simulink model "gm_parallel_phase_voltages_per_switching_state_6_vnl"  (R2022a)
settings: Solver=FixedStepDiscrete  StartTime=0.0  StopTime=10.0  RelTol=1e-3
undefined symbols (not defined in the file or in its folder): f_c, Rt, u_dc
libraries: hdlmdlgenlib x82, simulink x6, hdlsllib x2
(part 6 of 7)

== system gm_parallel_phase_voltages_per_switching_state_6_vnl/Phase_voltages_per_switching_state/Subsystem/MATLAB Function5/adder2 ==
  In1 : Inport
  In2 : Inport  Port=2
  adder2 : Sum  OutDataTypeStr=single  SampleTime=1e-08
  adder2_pd1 : Delay  DelayLength=6
  Out1 : Outport
  wires:
  adder2_pd1/1 -> Out1/1
  adder2/1 -> adder2_pd1/1
  In2/1 -> adder2/2
  In1/1 -> adder2/1

== system gm_parallel_phase_voltages_per_switching_state_6_vnl/Phase_voltages_per_switching_state/Subsystem/MATLAB Function5/cos_to_sincos ==
  In1 : Inport
  cos_to_sincos : Trigonometry  Operator=sincos  SampleTime=1e-08
  cos_to_sincos_pd1 : Delay  DelayLength=27
  cos_to_sincos_pd2 : Delay  DelayLength=27
  Out1 : Outport
  Out2 : Outport  Port=2
  wires:
  cos_to_sincos_pd2/1 -> Out2/1
  cos_to_sincos/2 -> cos_to_sincos_pd2/1
  cos_to_sincos_pd1/1 -> Out1/1
  cos_to_sincos/1 -> cos_to_sincos_pd1/1
  In1/1 -> cos_to_sincos/1

== system gm_parallel_phase_voltages_per_switching_state_6_vnl/Phase_voltages_per_switching_state/Subsystem/MATLAB Function5/multiplier ==
  In1 : Inport
  In2 : Inport  Port=2
  multiplier : Product  Inputs=**  OutDataTypeStr=single  SampleTime=1e-08
  multiplier_pd1 : Delay  DelayLength=6
  Out1 : Outport
  wires:
  multiplier_pd1/1 -> Out1/1
  multiplier/1 -> multiplier_pd1/1
  In2/1 -> multiplier/2
  In1/1 -> multiplier/1

== system gm_parallel_phase_voltages_per_switching_state_6_vnl/Phase_voltages_per_switching_state/Subsystem/MATLAB Function5/multiplier1 ==
  In1 : Inport
  In2 : Inport  Port=2
  multiplier1 : Product  Inputs=**  OutDataTypeStr=single  SampleTime=1e-08
  multiplier1_pd1 : Delay  DelayLength=6
  Out1 : Outport
  wires:
  multiplier1_pd1/1 -> Out1/1
  multiplier1/1 -> multiplier1_pd1/1
  In2/1 -> multiplier1/2
  In1/1 -> multiplier1/1

== system gm_parallel_phase_voltages_per_switching_state_6_vnl/Phase_voltages_per_switching_state/Subsystem/MATLAB Function5/multiplier2 ==
  In1 : Inport
  In2 : Inport  Port=2
  multiplier2 : Product  Inputs=**  OutDataTypeStr=single  SampleTime=1e-08
  multiplier2_pd1 : Delay  DelayLength=6
  Out1 : Outport
  wires:
  multiplier2_pd1/1 -> Out1/1
  multiplier2/1 -> multiplier2_pd1/1
  In2/1 -> multiplier2/2
  In1/1 -> multiplier2/1

== system gm_parallel_phase_voltages_per_switching_state_6_vnl/Phase_voltages_per_switching_state/Subsystem/MATLAB Function5/multiplier3 ==
  In1 : Inport
  In2 : Inport  Port=2
  multiplier3 : Product  Inputs=**  OutDataTypeStr=single  SampleTime=1e-08
  multiplier3_pd1 : Delay  DelayLength=6
  Out1 : Outport
  wires:
  multiplier3_pd1/1 -> Out1/1
  multiplier3/1 -> multiplier3_pd1/1
  In2/1 -> multiplier3/2
  In1/1 -> multiplier3/1

== system gm_parallel_phase_voltages_per_switching_state_6_vnl/Phase_voltages_per_switching_state/Subsystem/MATLAB Function5/multiplier4 ==
  In1 : Inport
  In2 : Inport  Port=2
  multiplier4 : Product  Inputs=**  OutDataTypeStr=single  SampleTime=1e-08
  multiplier4_pd1 : Delay  DelayLength=6
  Out1 : Outport
  wires:
  multiplier4_pd1/1 -> Out1/1
  multiplier4/1 -> multiplier4_pd1/1
  In2/1 -> multiplier4/2
  In1/1 -> multiplier4/1

== system gm_parallel_phase_voltages_per_switching_state_6_vnl/Phase_voltages_per_switching_state/Subsystem/MATLAB Function5/uminus ==
  In1 : Inport
  uminus : UnaryMinus  SampleTime=1e-08
  Out1 : Outport
  wires:
  uminus/1 -> Out1/1
  In1/1 -> uminus/1

== system gm_parallel_phase_voltages_per_switching_state_6_vnl/Phase_voltages_per_switching_state/Subsystem/MATLAB Function6/adder1 ==
  In1 : Inport
  In2 : Inport  Port=2
  adder1 : Sum  OutDataTypeStr=single  SampleTime=1e-08
  adder1_pd1 : Delay  DelayLength=6
  Out1 : Outport
  wires:
  adder1_pd1/1 -> Out1/1
  adder1/1 -> adder1_pd1/1
  In2/1 -> adder1/2
  In1/1 -> adder1/1

== system gm_parallel_phase_voltages_per_switching_state_6_vnl/Phase_voltages_per_switching_state/Subsystem/MATLAB Function6/adder2 ==
  In1 : Inport
  In2 : Inport  Port=2
  adder2 : Sum  OutDataTypeStr=single  SampleTime=1e-08
  adder2_pd1 : Delay  DelayLength=6
  Out1 : Outport
  wires:
  adder2_pd1/1 -> Out1/1
  adder2/1 -> adder2_pd1/1
  In2/1 -> adder2/2
  In1/1 -> adder2/1

== system gm_parallel_phase_voltages_per_switching_state_6_vnl/Phase_voltages_per_switching_state/Subsystem/MATLAB Function6/cos_to_sincos ==
  In1 : Inport
  cos_to_sincos : Trigonometry  Operator=sincos  SampleTime=1e-08
  cos_to_sincos_pd1 : Delay  DelayLength=27
  cos_to_sincos_pd2 : Delay  DelayLength=27
  Out1 : Outport
  Out2 : Outport  Port=2
  wires:
  cos_to_sincos_pd2/1 -> Out2/1
  cos_to_sincos/2 -> cos_to_sincos_pd2/1
  cos_to_sincos_pd1/1 -> Out1/1
  cos_to_sincos/1 -> cos_to_sincos_pd1/1
  In1/1 -> cos_to_sincos/1

== system gm_parallel_phase_voltages_per_switching_state_6_vnl/Phase_voltages_per_switching_state/Subsystem/MATLAB Function6/multiplier ==
  In1 : Inport
  In2 : Inport  Port=2
  multiplier : Product  Inputs=**  OutDataTypeStr=single  SampleTime=1e-08
  multiplier_pd1 : Delay  DelayLength=6
  Out1 : Outport
  wires:
  multiplier_pd1/1 -> Out1/1
  multiplier/1 -> multiplier_pd1/1
  In2/1 -> multiplier/2
  In1/1 -> multiplier/1

== system gm_parallel_phase_voltages_per_switching_state_6_vnl/Phase_voltages_per_switching_state/Subsystem/MATLAB Function6/multiplier1 ==
  In1 : Inport
  In2 : Inport  Port=2
  multiplier1 : Product  Inputs=**  OutDataTypeStr=single  SampleTime=1e-08
  multiplier1_pd1 : Delay  DelayLength=6
  Out1 : Outport
  wires:
  multiplier1_pd1/1 -> Out1/1
  multiplier1/1 -> multiplier1_pd1/1
  In2/1 -> multiplier1/2
  In1/1 -> multiplier1/1

== system gm_parallel_phase_voltages_per_switching_state_6_vnl/Phase_voltages_per_switching_state/Subsystem/MATLAB Function6/multiplier2 ==
  In1 : Inport
  In2 : Inport  Port=2
  multiplier2 : Product  Inputs=**  OutDataTypeStr=single  SampleTime=1e-08
  multiplier2_pd1 : Delay  DelayLength=6
  Out1 : Outport
  wires:
  multiplier2_pd1/1 -> Out1/1
  multiplier2/1 -> multiplier2_pd1/1
  In2/1 -> multiplier2/2
  In1/1 -> multiplier2/1

== system gm_parallel_phase_voltages_per_switching_state_6_vnl/Phase_voltages_per_switching_state/Subsystem/MATLAB Function6/multiplier3 ==
  In1 : Inport
  In2 : Inport  Port=2
  multiplier3 : Product  Inputs=**  OutDataTypeStr=single  SampleTime=1e-08
  multiplier3_pd1 : Delay  DelayLength=6
  Out1 : Outport
  wires:
  multiplier3_pd1/1 -> Out1/1
  multiplier3/1 -> multiplier3_pd1/1
  In2/1 -> multiplier3/2
  In1/1 -> multiplier3/1

== system gm_parallel_phase_voltages_per_switching_state_6_vnl/Phase_voltages_per_switching_state/Subsystem/MATLAB Function6/multiplier4 ==
  In1 : Inport
  In2 : Inport  Port=2
  multiplier4 : Product  Inputs=**  OutDataTypeStr=single  SampleTime=1e-08
  multiplier4_pd1 : Delay  DelayLength=6
  Out1 : Outport
  wires:
  multiplier4_pd1/1 -> Out1/1
  multiplier4/1 -> multiplier4_pd1/1
  In2/1 -> multiplier4/2
  In1/1 -> multiplier4/1

== system gm_parallel_phase_voltages_per_switching_state_6_vnl/Phase_voltages_per_switching_state/Subsystem/MATLAB Function6/uminus ==
  In1 : Inport
  uminus : UnaryMinus  SampleTime=1e-08
  Out1 : Outport
  wires:
  uminus/1 -> Out1/1
  In1/1 -> uminus/1

== system gm_parallel_phase_voltages_per_switching_state_6_vnl/Phase_voltages_per_switching_state/Subsystem/MATLAB Function7/adder1 ==
  In1 : Inport
  In2 : Inport  Port=2
  adder1 : Sum  OutDataTypeStr=single  SampleTime=1e-08
  adder1_pd1 : Delay  DelayLength=6
  Out1 : Outport
  wires:
  adder1_pd1/1 -> Out1/1
  adder1/1 -> adder1_pd1/1
  In2/1 -> adder1/2
  In1/1 -> adder1/1

== system gm_parallel_phase_voltages_per_switching_state_6_vnl/Phase_voltages_per_switching_state/Subsystem/MATLAB Function7/adder2 ==
  In1 : Inport
  In2 : Inport  Port=2
  adder2 : Sum  OutDataTypeStr=single  SampleTime=1e-08
  adder2_pd1 : Delay  DelayLength=6
  Out1 : Outport
  wires:
  adder2_pd1/1 -> Out1/1
  adder2/1 -> adder2_pd1/1
  In2/1 -> adder2/2
  In1/1 -> adder2/1

== system gm_parallel_phase_voltages_per_switching_state_6_vnl/Phase_voltages_per_switching_state/Subsystem/MATLAB Function7/cos_to_sincos ==
  In1 : Inport
  cos_to_sincos : Trigonometry  Operator=sincos  SampleTime=1e-08
  cos_to_sincos_pd1 : Delay  DelayLength=27
  cos_to_sincos_pd2 : Delay  DelayLength=27
  Out1 : Outport
  Out2 : Outport  Port=2
  wires:
  cos_to_sincos_pd2/1 -> Out2/1
  cos_to_sincos/2 -> cos_to_sincos_pd2/1
  cos_to_sincos_pd1/1 -> Out1/1
  cos_to_sincos/1 -> cos_to_sincos_pd1/1
  In1/1 -> cos_to_sincos/1

== system gm_parallel_phase_voltages_per_switching_state_6_vnl/Phase_voltages_per_switching_state/Subsystem/MATLAB Function7/multiplier ==
  In1 : Inport
  In2 : Inport  Port=2
  multiplier : Product  Inputs=**  OutDataTypeStr=single  SampleTime=1e-08
  multiplier_pd1 : Delay  DelayLength=6
  Out1 : Outport
  wires:
  multiplier_pd1/1 -> Out1/1
  multiplier/1 -> multiplier_pd1/1
  In2/1 -> multiplier/2
  In1/1 -> multiplier/1

== system gm_parallel_phase_voltages_per_switching_state_6_vnl/Phase_voltages_per_switching_state/Subsystem/MATLAB Function7/multiplier1 ==
  In1 : Inport
  In2 : Inport  Port=2
  multiplier1 : Product  Inputs=**  OutDataTypeStr=single  SampleTime=1e-08
  multiplier1_pd1 : Delay  DelayLength=6
  Out1 : Outport
  wires:
  multiplier1_pd1/1 -> Out1/1
  multiplier1/1 -> multiplier1_pd1/1
  In2/1 -> multiplier1/2
  In1/1 -> multiplier1/1

== system gm_parallel_phase_voltages_per_switching_state_6_vnl/Phase_voltages_per_switching_state/Subsystem/MATLAB Function7/multiplier2 ==
  In1 : Inport
  In2 : Inport  Port=2
  multiplier2 : Product  Inputs=**  OutDataTypeStr=single  SampleTime=1e-08
  multiplier2_pd1 : Delay  DelayLength=6
  Out1 : Outport
  wires:
  multiplier2_pd1/1 -> Out1/1
  multiplier2/1 -> multiplier2_pd1/1
  In2/1 -> multiplier2/2
  In1/1 -> multiplier2/1

== system gm_parallel_phase_voltages_per_switching_state_6_vnl/Phase_voltages_per_switching_state/Subsystem/MATLAB Function7/multiplier3 ==
  In1 : Inport
  In2 : Inport  Port=2
  multiplier3 : Product  Inputs=**  OutDataTypeStr=single  SampleTime=1e-08
  multiplier3_pd1 : Delay  DelayLength=6
  Out1 : Outport
  wires:
  multiplier3_pd1/1 -> Out1/1
  multiplier3/1 -> multiplier3_pd1/1
  In2/1 -> multiplier3/2
  In1/1 -> multiplier3/1

== system gm_parallel_phase_voltages_per_switching_state_6_vnl/Phase_voltages_per_switching_state/Subsystem/MATLAB Function7/multiplier4 ==
  In1 : Inport
  In2 : Inport  Port=2
  multiplier4 : Product  Inputs=**  OutDataTypeStr=single  SampleTime=1e-08
  multiplier4_pd1 : Delay  DelayLength=6
  Out1 : Outport
  wires:
  multiplier4_pd1/1 -> Out1/1
  multiplier4/1 -> multiplier4_pd1/1
  In2/1 -> multiplier4/2
  In1/1 -> multiplier4/1

== system gm_parallel_phase_voltages_per_switching_state_6_vnl/Phase_voltages_per_switching_state/Subsystem/MATLAB Function7/uminus ==
  In1 : Inport
  uminus : UnaryMinus  SampleTime=1e-08
  Out1 : Outport
  wires:
  uminus/1 -> Out1/1
  In1/1 -> uminus/1

== system gm_parallel_phase_voltages_per_switching_state_6_vnl/Phase_voltages_per_switching_state/Subsystem/MATLAB Function8/adder1 ==
  In1 : Inport
  In2 : Inport  Port=2
  adder1 : Sum  OutDataTypeStr=single  SampleTime=1e-08
  adder1_pd1 : Delay  DelayLength=6
  Out1 : Outport
  wires:
  adder1_pd1/1 -> Out1/1
  adder1/1 -> adder1_pd1/1
  In2/1 -> adder1/2
  In1/1 -> adder1/1

== system gm_parallel_phase_voltages_per_switching_state_6_vnl/Phase_voltages_per_switching_state/Subsystem/MATLAB Function8/adder2 ==
  In1 : Inport
  In2 : Inport  Port=2
  adder2 : Sum  OutDataTypeStr=single  SampleTime=1e-08
  adder2_pd1 : Delay  DelayLength=6
  Out1 : Outport
  wires:
  adder2_pd1/1 -> Out1/1
  adder2/1 -> adder2_pd1/1
  In2/1 -> adder2/2
  In1/1 -> adder2/1

== system gm_parallel_phase_voltages_per_switching_state_6_vnl/Phase_voltages_per_switching_state/Subsystem/MATLAB Function8/cos_to_sincos ==
  In1 : Inport
  cos_to_sincos : Trigonometry  Operator=sincos  SampleTime=1e-08
  cos_to_sincos_pd1 : Delay  DelayLength=27
  cos_to_sincos_pd2 : Delay  DelayLength=27
  Out1 : Outport
  Out2 : Outport  Port=2
  wires:
  cos_to_sincos_pd2/1 -> Out2/1
  cos_to_sincos/2 -> cos_to_sincos_pd2/1
  cos_to_sincos_pd1/1 -> Out1/1
  cos_to_sincos/1 -> cos_to_sincos_pd1/1
  In1/1 -> cos_to_sincos/1

== system gm_parallel_phase_voltages_per_switching_state_6_vnl/Phase_voltages_per_switching_state/Subsystem/MATLAB Function8/multiplier ==
  In1 : Inport
  In2 : Inport  Port=2
  multiplier : Product  Inputs=**  OutDataTypeStr=single  SampleTime=1e-08
  multiplier_pd1 : Delay  DelayLength=6
  Out1 : Outport
  wires:
  multiplier_pd1/1 -> Out1/1
  multiplier/1 -> multiplier_pd1/1
  In2/1 -> multiplier/2
  In1/1 -> multiplier/1

== system gm_parallel_phase_voltages_per_switching_state_6_vnl/Phase_voltages_per_switching_state/Subsystem/MATLAB Function8/multiplier1 ==
  In1 : Inport
  In2 : Inport  Port=2
  multiplier1 : Product  Inputs=**  OutDataTypeStr=single  SampleTime=1e-08
  multiplier1_pd1 : Delay  DelayLength=6
  Out1 : Outport
  wires:
  multiplier1_pd1/1 -> Out1/1
  multiplier1/1 -> multiplier1_pd1/1
  In2/1 -> multiplier1/2
  In1/1 -> multiplier1/1

== system gm_parallel_phase_voltages_per_switching_state_6_vnl/Phase_voltages_per_switching_state/Subsystem/MATLAB Function8/multiplier2 ==
  In1 : Inport
  In2 : Inport  Port=2
  multiplier2 : Product  Inputs=**  OutDataTypeStr=single  SampleTime=1e-08
  multiplier2_pd1 : Delay  DelayLength=6
  Out1 : Outport
  wires:
  multiplier2_pd1/1 -> Out1/1
  multiplier2/1 -> multiplier2_pd1/1
  In2/1 -> multiplier2/2
  In1/1 -> multiplier2/1

== system gm_parallel_phase_voltages_per_switching_state_6_vnl/Phase_voltages_per_switching_state/Subsystem/MATLAB Function8/multiplier3 ==
  In1 : Inport
  In2 : Inport  Port=2
  multiplier3 : Product  Inputs=**  OutDataTypeStr=single  SampleTime=1e-08
  multiplier3_pd1 : Delay  DelayLength=6
  Out1 : Outport
  wires:
  multiplier3_pd1/1 -> Out1/1
  multiplier3/1 -> multiplier3_pd1/1
  In2/1 -> multiplier3/2
  In1/1 -> multiplier3/1

== system gm_parallel_phase_voltages_per_switching_state_6_vnl/Phase_voltages_per_switching_state/Subsystem/MATLAB Function8/multiplier4 ==
  In1 : Inport
  In2 : Inport  Port=2
  multiplier4 : Product  Inputs=**  OutDataTypeStr=single  SampleTime=1e-08
  multiplier4_pd1 : Delay  DelayLength=6
  Out1 : Outport
  wires:
  multiplier4_pd1/1 -> Out1/1
  multiplier4/1 -> multiplier4_pd1/1
  In2/1 -> multiplier4/2
  In1/1 -> multiplier4/1

== system gm_parallel_phase_voltages_per_switching_state_6_vnl/Phase_voltages_per_switching_state/Subsystem/MATLAB Function8/uminus ==
  In1 : Inport
  uminus : UnaryMinus  SampleTime=1e-08
  Out1 : Outport
  wires:
  uminus/1 -> Out1/1
  In1/1 -> uminus/1

== system gm_parallel_phase_voltages_per_switching_state_6_vnl/Phase_voltages_per_switching_state/Subsystem/MATLAB Function9/adder1 ==
  In1 : Inport
  In2 : Inport  Port=2
  adder1 : Sum  OutDataTypeStr=single  SampleTime=1e-08
  adder1_pd1 : Delay  DelayLength=6
  Out1 : Outport
  wires:
  adder1_pd1/1 -> Out1/1
  adder1/1 -> adder1_pd1/1
  In2/1 -> adder1/2
  In1/1 -> adder1/1

== system gm_parallel_phase_voltages_per_switching_state_6_vnl/Phase_voltages_per_switching_state/Subsystem/MATLAB Function9/adder2 ==
  In1 : Inport
  In2 : Inport  Port=2
  adder2 : Sum  OutDataTypeStr=single  SampleTime=1e-08
  adder2_pd1 : Delay  DelayLength=6
  Out1 : Outport
  wires:
  adder2_pd1/1 -> Out1/1
  adder2/1 -> adder2_pd1/1
  In2/1 -> adder2/2
  In1/1 -> adder2/1

== system gm_parallel_phase_voltages_per_switching_state_6_vnl/Phase_voltages_per_switching_state/Subsystem/MATLAB Function9/cos_to_sincos ==
  In1 : Inport
  cos_to_sincos : Trigonometry  Operator=sincos  SampleTime=1e-08
  cos_to_sincos_pd1 : Delay  DelayLength=27
  cos_to_sincos_pd2 : Delay  DelayLength=27
  Out1 : Outport
  Out2 : Outport  Port=2
  wires:
  cos_to_sincos_pd2/1 -> Out2/1
  cos_to_sincos/2 -> cos_to_sincos_pd2/1
  cos_to_sincos_pd1/1 -> Out1/1
  cos_to_sincos/1 -> cos_to_sincos_pd1/1
  In1/1 -> cos_to_sincos/1

== system gm_parallel_phase_voltages_per_switching_state_6_vnl/Phase_voltages_per_switching_state/Subsystem/MATLAB Function9/multiplier ==
  In1 : Inport
  In2 : Inport  Port=2
  multiplier : Product  Inputs=**  OutDataTypeStr=single  SampleTime=1e-08
  multiplier_pd1 : Delay  DelayLength=6
  Out1 : Outport
  wires:
  multiplier_pd1/1 -> Out1/1
  multiplier/1 -> multiplier_pd1/1
  In2/1 -> multiplier/2
  In1/1 -> multiplier/1

== system gm_parallel_phase_voltages_per_switching_state_6_vnl/Phase_voltages_per_switching_state/Subsystem/MATLAB Function9/multiplier1 ==
  In1 : Inport
  In2 : Inport  Port=2
  multiplier1 : Product  Inputs=**  OutDataTypeStr=single  SampleTime=1e-08
  multiplier1_pd1 : Delay  DelayLength=6
  Out1 : Outport
  wires:
  multiplier1_pd1/1 -> Out1/1
  multiplier1/1 -> multiplier1_pd1/1
  In2/1 -> multiplier1/2
  In1/1 -> multiplier1/1

== system gm_parallel_phase_voltages_per_switching_state_6_vnl/Phase_voltages_per_switching_state/Subsystem/MATLAB Function9/multiplier2 ==
  In1 : Inport
  In2 : Inport  Port=2
  multiplier2 : Product  Inputs=**  OutDataTypeStr=single  SampleTime=1e-08
  multiplier2_pd1 : Delay  DelayLength=6
  Out1 : Outport
  wires:
  multiplier2_pd1/1 -> Out1/1
  multiplier2/1 -> multiplier2_pd1/1
  In2/1 -> multiplier2/2
  In1/1 -> multiplier2/1

== system gm_parallel_phase_voltages_per_switching_state_6_vnl/Phase_voltages_per_switching_state/Subsystem/MATLAB Function9/multiplier3 ==
  In1 : Inport
  In2 : Inport  Port=2
  multiplier3 : Product  Inputs=**  OutDataTypeStr=single  SampleTime=1e-08
  multiplier3_pd1 : Delay  DelayLength=6
  Out1 : Outport
  wires:
  multiplier3_pd1/1 -> Out1/1
  multiplier3/1 -> multiplier3_pd1/1
  In2/1 -> multiplier3/2
  In1/1 -> multiplier3/1

== system gm_parallel_phase_voltages_per_switching_state_6_vnl/Phase_voltages_per_switching_state/Subsystem/MATLAB Function9/multiplier4 ==
  In1 : Inport
  In2 : Inport  Port=2
  multiplier4 : Product  Inputs=**  OutDataTypeStr=single  SampleTime=1e-08
  multiplier4_pd1 : Delay  DelayLength=6
  Out1 : Outport
  wires:
  multiplier4_pd1/1 -> Out1/1
  multiplier4/1 -> multiplier4_pd1/1
  In2/1 -> multiplier4/2
  In1/1 -> multiplier4/1

== system gm_parallel_phase_voltages_per_switching_state_6_vnl/Phase_voltages_per_switching_state/Subsystem/MATLAB Function9/uminus ==
  In1 : Inport
  uminus : UnaryMinus  SampleTime=1e-08
  Out1 : Outport
  wires:
  uminus/1 -> Out1/1
  In1/1 -> uminus/1

== matlab function gm_parallel_phase_voltages_per_switching_state_6_vnl/Phase_voltages_per_switching_state_vnl/Subsystem/MATLAB Function8 ==
  data: theta_el_with_offset input; d_voltage_per_switching_state output; u_dc_link_voltage input; Index input; q_voltage_per_switching_state output; x_voltage_per_switching_state output; y_voltage_per_switching_state output
function [d_voltage_per_switching_state, q_voltage_per_switching_state, x_voltage_per_switching_state, y_voltage_per_switching_state] = fcn(theta_el_with_offset, u_dc_link_voltage, Index)
      
        % Initial condition
            Index = Index+1;

    
        % Swichtingstates factors alpha beta x y
        Factors_alpha_beta_x_y = single([-0.166666666666667	 0.166666666666667	 -0.333333333333333	0;
                                         0.0446581987385205	 0.0446581987385205	  0.333333333333333	0.333333333333333;
                                         -0.166666666666667	 0.166666666666667	 -0.333333333333333	0;
                                         0.622008467928146	 0.622008467928146	  0.333333333333333	0.333333333333333]);
        
        % Park-Transformation of the switchingstates factors
        Factors_d_q_x_y =single(zeros(4,1));
    
        Factors_d_q_x_y(3,1) = Factors_alpha_beta_x_y(3,Index);
        Factors_d_q_x_y(4,1) = Factors_alpha_beta_x_y(4,Index);
    
        cos_theta_el = single(cos(theta_el_with_offset));
        sin_theta_el = single(sin(theta_el_with_offset));
       
        Factors_d_q_x_y(1,1) = cos_theta_el*Factors_alpha_beta_x_y(1,Index)+sin_theta_el*Factors_alpha_beta_x_y(2,Index);
        Factors_d_q_x_y(2,1) = -sin_theta_el*Factors_alpha_beta_x_y(1,Index)+cos_theta_el*Factors_alpha_beta_x_y(2,Index);
    
        %Calculation of the voltages per switching state in alpha beta coordinates
        d_q_x_y_voltages_per_switching_state = single(u_dc_link_voltage*Factors_d_q_x_y);
    
        d_voltage_per_switching_state = d_q_x_y_voltages_per_switching_state(1,1);
        q_voltage_per_switching_state = d_q_x_y_voltages_per_switching_state(2,1);
        x_voltage_per_switching_state = d_q_x_y_voltages_per_switching_state(3,1);
        y_voltage_per_switching_state = d_q_x_y_voltages_per_switching_state(4,1);
    

end

== matlab function gm_parallel_phase_voltages_per_switching_state_6_vnl/Phase_voltages_per_switching_state_vnl/Subsystem/MATLAB Function9 ==
  data: theta_el_with_offset input; d_voltage_per_switching_state output; u_dc_link_voltage input; Index input; q_voltage_per_switching_state output; x_voltage_per_switching_state output; y_voltage_per_switching_state output
function [d_voltage_per_switching_state, q_voltage_per_switching_state, x_voltage_per_switching_state, y_voltage_per_switching_state] = fcn(theta_el_with_offset, u_dc_link_voltage, Index)
      
        % Initial condition
            Index = Index+1;

    
        % Swichtingstates factors alpha beta x y
        Factors_alpha_beta_x_y = single([0	                0.333333333333333	-0.166666666666667  	0.166666666666667;
                                         0.333333333333333	0.333333333333333	 0.622008467928146	    0.622008467928146;
                                         0	                0.333333333333333	-0.166666666666667	    0.166666666666667;
                                         0.333333333333333	0.333333333333333	 0.0446581987385205 	0.0446581987385205]);
        
        % Park-Transformation of the switchingstates factors
        Factors_d_q_x_y =single(zeros(4,1));
    
        Factors_d_q_x_y(3,1) = Factors_alpha_beta_x_y(3,Index);
        Factors_d_q_x_y(4,1) = Factors_alpha_beta_x_y(4,Index);
    
        cos_theta_el = single(cos(theta_el_with_offset));
        sin_theta_el = single(sin(theta_el_with_offset));
       
        Factors_d_q_x_y(1,1) = cos_theta_el*Factors_alpha_beta_x_y(1,Index)+sin_theta_el*Factors_alpha_beta_x_y(2,Index);
        Factors_d_q_x_y(2,1) = -sin_theta_el*Factors_alpha_beta_x_y(1,Index)+cos_theta_el*Factors_alpha_beta_x_y(2,Index);
    
        %Calculation of the voltages per switching state in alpha beta coordinates
        d_q_x_y_voltages_per_switching_state = single(u_dc_link_voltage*Factors_d_q_x_y);
    
        d_voltage_per_switching_state = d_q_x_y_voltages_per_switching_state(1,1);
        q_voltage_per_switching_state = d_q_x_y_voltages_per_switching_state(2,1);
        x_voltage_per_switching_state = d_q_x_y_voltages_per_switching_state(3,1);
        y_voltage_per_switching_state = d_q_x_y_voltages_per_switching_state(4,1);
    

end

== matlab function gm_parallel_phase_voltages_per_switching_state_6_vnl/Phase_voltages_per_switching_state_vnl/Subsystem/MATLAB Function10 ==
  data: theta_el_with_offset input; d_voltage_per_switching_state output; u_dc_link_voltage input; Index input; q_voltage_per_switching_state output; x_voltage_per_switching_state output; y_voltage_per_switching_state output
function [d_voltage_per_switching_state, q_voltage_per_switching_state, x_voltage_per_switching_state, y_voltage_per_switching_state] = fcn(theta_el_with_offset, u_dc_link_voltage, Index)
      
        % Initial condition
            Index = Index+1;

        % Swichtingstates factors alpha beta x y
        Factors_alpha_beta_x_y = single([-0.455341801261480	-0.122008467928146	-0.622008467928146	-0.288675134594813;
                                         -0.122008467928146	-0.122008467928146	 0.166666666666667	 0.166666666666667;
                                          0.122008467928146	 0.455341801261480	-0.0446581987385205	 0.288675134594813;
                                          0.455341801261480	 0.455341801261480	 0.166666666666667	 0.166666666666667]);
        
        % Park-Transformation of the switchingstates factors
        Factors_d_q_x_y =single(zeros(4,1));
    
        Factors_d_q_x_y(3,1) = Factors_alpha_beta_x_y(3,Index);
        Factors_d_q_x_y(4,1) = Factors_alpha_beta_x_y(4,Index);
    
        cos_theta_el = single(cos(theta_el_with_offset));
        sin_theta_el = single(sin(theta_el_with_offset));
       
        Factors_d_q_x_y(1,1) = cos_theta_el*Factors_alpha_beta_x_y(1,Index)+sin_theta_el*Factors_alpha_beta_x_y(2,Index);
        Factors_d_q_x_y(2,1) = -sin_theta_el*Factors_alpha_beta_x_y(1,Index)+cos_theta_el*Factors_alpha_beta_x_y(2,Index);
    
        %Calculation of the voltages per switching state in alpha beta coordinates
        d_q_x_y_voltages_per_switching_state = single(u_dc_link_voltage*Factors_d_q_x_y);
    
        d_voltage_per_switching_state = d_q_x_y_voltages_per_switching_state(1,1);
        q_voltage_per_switching_state = d_q_x_y_voltages_per_switching_state(2,1);
        x_voltage_per_switching_state = d_q_x_y_voltages_per_switching_state(3,1);
        y_voltage_per_switching_state = d_q_x_y_voltages_per_switching_state(4,1);
    

end

== matlab function gm_parallel_phase_voltages_per_switching_state_6_vnl/Phase_voltages_per_switching_state_vnl/Subsystem/MATLAB Function ==
  data: theta_el_with_offset input; d_voltage_per_switching_state output; u_dc_link_voltage input; Index input; q_voltage_per_switching_state output; x_voltage_per_switching_state output; y_voltage_per_switching_state output
function [d_voltage_per_switching_state, q_voltage_per_switching_state, x_voltage_per_switching_state, y_voltage_per_switching_state] = fcn(theta_el_with_offset, u_dc_link_voltage, Index)
      
        % Initial condition
            Index = Index+1;

    
        % Swichtingstates factors alpha beta x y
        Factors_alpha_beta_x_y = single([-0.166666666666667	 0.166666666666667	-0.333333333333333	0;
                                         -0.288675134594813	-0.288675134594813	 0	                0;
                                         -0.166666666666667	 0.166666666666667	-0.333333333333333	0;
                                         0.288675134594813	 0.288675134594813	 0	                0]);
        
        % Park-Transformation of the switchingstates factors
        Factors_d_q_x_y =single(zeros(4,1));
    
        Factors_d_q_x_y(3,1) = Factors_alpha_beta_x_y(3,Index);
        Factors_d_q_x_y(4,1) = Factors_alpha_beta_x_y(4,Index);
    
        cos_theta_el = single(cos(theta_el_with_offset));
        sin_theta_el = single(sin(theta_el_with_offset));
       
        Factors_d_q_x_y(1,1) = cos_theta_el*Factors_alpha_beta_x_y(1,Index)+sin_theta_el*Factors_alpha_beta_x_y(2,Index);
        Factors_d_q_x_y(2,1) = -sin_theta_el*Factors_alpha_beta_x_y(1,Index)+cos_theta_el*Factors_alpha_beta_x_y(2,Index);
    
        %Calculation of the voltages per switching state in alpha beta coordinates
        d_q_x_y_voltages_per_switching_state = single(u_dc_link_voltage*Factors_d_q_x_y);
    
        d_voltage_per_switching_state = d_q_x_y_voltages_per_switching_state(1,1);
        q_voltage_per_switching_state = d_q_x_y_voltages_per_switching_state(2,1);
        x_voltage_per_switching_state = d_q_x_y_voltages_per_switching_state(3,1);
        y_voltage_per_switching_state = d_q_x_y_voltages_per_switching_state(4,1);
    

end

== matlab function gm_parallel_phase_voltages_per_switching_state_6_vnl/Phase_voltages_per_switching_state_vnl/Subsystem/MATLAB Function11 ==
  data: theta_el_with_offset input; d_voltage_per_switching_state output; u_dc_link_voltage input; Index input; q_voltage_per_switching_state output; x_voltage_per_switching_state output; y_voltage_per_switching_state output
function [d_voltage_per_switching_state, q_voltage_per_switching_state, x_voltage_per_switching_state, y_voltage_per_switching_state] = fcn(theta_el_with_offset, u_dc_link_voltage, Index)
      
        % Initial condition
            Index = Index+1;

    
        % Swichtingstates factors alpha beta x y
        Factors_alpha_beta_x_y = single([-0.288675134594813	0.0446581987385205	-0.455341801261480	-0.122008467928146;
                                         0.166666666666667	0.166666666666667	 0.455341801261480   0.455341801261480;
                                         0.288675134594813	0.622008467928146	 0.122008467928146	 0.455341801261480;
                                         0.166666666666667	0.166666666666667	-0.122008467928146	-0.122008467928146]);
        
        % Park-Transformation of the switchingstates factors
        Factors_d_q_x_y =single(zeros(4,1));
    
        Factors_d_q_x_y(3,1) = Factors_alpha_beta_x_y(3,Index);
        Factors_d_q_x_y(4,1) = Factors_alpha_beta_x_y(4,Index);
    
        cos_theta_el = single(cos(theta_el_with_offset));
        sin_theta_el = single(sin(theta_el_with_offset));
       
        Factors_d_q_x_y(1,1) = cos_theta_el*Factors_alpha_beta_x_y(1,Index)+sin_theta_el*Factors_alpha_beta_x_y(2,Index);
        Factors_d_q_x_y(2,1) = -sin_theta_el*Factors_alpha_beta_x_y(1,Index)+cos_theta_el*Factors_alpha_beta_x_y(2,Index);
    
        %Calculation of the voltages per switching state in alpha beta coordinates
        d_q_x_y_voltages_per_switching_state = single(u_dc_link_voltage*Factors_d_q_x_y);
    
        d_voltage_per_switching_state = d_q_x_y_voltages_per_switching_state(1,1);
        q_voltage_per_switching_state = d_q_x_y_voltages_per_switching_state(2,1);
        x_voltage_per_switching_state = d_q_x_y_voltages_per_switching_state(3,1);
        y_voltage_per_switching_state = d_q_x_y_voltages_per_switching_state(4,1);
    

end

== matlab function gm_parallel_phase_voltages_per_switching_state_6_vnl/Phase_voltages_per_switching_state_vnl/Subsystem/MATLAB Function12 ==
  data: theta_el_with_offset input; d_voltage_per_switching_state output; u_dc_link_voltage input; Index input; q_voltage_per_switching_state output; x_voltage_per_switching_state output; y_voltage_per_switching_state output
function [d_voltage_per_switching_state, q_voltage_per_switching_state, x_voltage_per_switching_state, y_voltage_per_switching_state] = fcn(theta_el_with_offset, u_dc_link_voltage, Index)
      
        % Initial condition
            Index = Index+1;

    
        % Swichtingstates factors alpha beta x y
        Factors_alpha_beta_x_y = single([0.122008467928146	 0.455341801261480	-0.0446581987385205  0.288675134594813;
                                        -0.122008467928146	-0.122008467928146	 0.166666666666667	 0.166666666666667;
                                        -0.455341801261480	-0.122008467928146	-0.622008467928146	-0.288675134594813;
                                         0.455341801261480	 0.455341801261480	 0.166666666666667	 0.166666666666667]);
        
        % Park-Transformation of the switchingstates factors
        Factors_d_q_x_y =single(zeros(4,1));
    
        Factors_d_q_x_y(3,1) = Factors_alpha_beta_x_y(3,Index);
        Factors_d_q_x_y(4,1) = Factors_alpha_beta_x_y(4,Index);
    
        cos_theta_el = single(cos(theta_el_with_offset));
        sin_theta_el = single(sin(theta_el_with_offset));
       
        Factors_d_q_x_y(1,1) = cos_theta_el*Factors_alpha_beta_x_y(1,Index)+sin_theta_el*Factors_alpha_beta_x_y(2,Index);
        Factors_d_q_x_y(2,1) = -sin_theta_el*Factors_alpha_beta_x_y(1,Index)+cos_theta_el*Factors_alpha_beta_x_y(2,Index);
    
        %Calculation of the voltages per switching state in alpha beta coordinates
        d_q_x_y_voltages_per_switching_state = single(u_dc_link_voltage*Factors_d_q_x_y);
    
        d_voltage_per_switching_state = d_q_x_y_voltages_per_switching_state(1,1);
        q_voltage_per_switching_state = d_q_x_y_voltages_per_switching_state(2,1);
        x_voltage_per_switching_state = d_q_x_y_voltages_per_switching_state(3,1);
        y_voltage_per_switching_state = d_q_x_y_voltages_per_switching_state(4,1);
    

end

== matlab function gm_parallel_phase_voltages_per_switching_state_6_vnl/Phase_voltages_per_switching_state_vnl/Subsystem/MATLAB Function13 ==
  data: theta_el_with_offset input; d_voltage_per_switching_state output; u_dc_link_voltage input; Index input; q_voltage_per_switching_state output; x_voltage_per_switching_state output; y_voltage_per_switching_state output
function [d_voltage_per_switching_state, q_voltage_per_switching_state, x_voltage_per_switching_state, y_voltage_per_switching_state] = fcn(theta_el_with_offset, u_dc_link_voltage, Index)
      
        % Initial condition
            Index = Index+1;

    
        % Swichtingstates factors alpha beta x y
        Factors_alpha_beta_x_y = single([0.288675134594813	0.622008467928146	 0.122008467928146  	0.455341801261480;
                                         0.166666666666667	0.166666666666667	 0.455341801261480  	0.455341801261480;
                                         -0.288675134594813	0.0446581987385205	-0.455341801261480	   -0.122008467928146;
                                         0.166666666666667	0.166666666666667	-0.122008467928146     -0.122008467928146]);
        
        % Park-Transformation of the switchingstates factors
        Factors_d_q_x_y =single(zeros(4,1));
    
        Factors_d_q_x_y(3,1) = Factors_alpha_beta_x_y(3,Index);
        Factors_d_q_x_y(4,1) = Factors_alpha_beta_x_y(4,Index);
    
        cos_theta_el = single(cos(theta_el_with_offset));
        sin_theta_el = single(sin(theta_el_with_offset));
       
        Factors_d_q_x_y(1,1) = cos_theta_el*Factors_alpha_beta_x_y(1,Index)+sin_theta_el*Factors_alpha_beta_x_y(2,Index);
        Factors_d_q_x_y(2,1) = -sin_theta_el*Factors_alpha_beta_x_y(1,Index)+cos_theta_el*Factors_alpha_beta_x_y(2,Index);
    
        %Calculation of the voltages per switching state in alpha beta coordinates
        d_q_x_y_voltages_per_switching_state = single(u_dc_link_voltage*Factors_d_q_x_y);
    
        d_voltage_per_switching_state = d_q_x_y_voltages_per_switching_state(1,1);
        q_voltage_per_switching_state = d_q_x_y_voltages_per_switching_state(2,1);
        x_voltage_per_switching_state = d_q_x_y_voltages_per_switching_state(3,1);
        y_voltage_per_switching_state = d_q_x_y_voltages_per_switching_state(4,1);
    

end

== matlab function gm_parallel_phase_voltages_per_switching_state_6_vnl/Phase_voltages_per_switching_state_vnl/Subsystem/MATLAB Function14 ==
  data: theta_el_with_offset input; d_voltage_per_switching_state output; u_dc_link_voltage input; Index input; q_voltage_per_switching_state output; x_voltage_per_switching_state output; y_voltage_per_switching_state output
function [d_voltage_per_switching_state, q_voltage_per_switching_state, x_voltage_per_switching_state, y_voltage_per_switching_state] = fcn(theta_el_with_offset, u_dc_link_voltage, Index)
      
        % Initial condition
            Index = Index+1;

    
        % Swichtingstates factors alpha beta x y
        Factors_alpha_beta_x_y = single([-0.166666666666667	 0.166666666666667	-0.333333333333333	0;
                                         -0.288675134594813	-0.288675134594813	 0	                0;
                                         -0.166666666666667	 0.166666666666667	-0.333333333333333	0;
                                          0.288675134594813	 0.288675134594813	 0              	0]);
        
        % Park-Transformation of the switchingstates factors
        Factors_d_q_x_y =single(zeros(4,1));
    
        Factors_d_q_x_y(3,1) = Factors_alpha_beta_x_y(3,Index);
        Factors_d_q_x_y(4,1) = Factors_alpha_beta_x_y(4,Index);
    
        cos_theta_el = single(cos(theta_el_with_offset));
        sin_theta_el = single(sin(theta_el_with_offset));
       
        Factors_d_q_x_y(1,1) = cos_theta_el*Factors_alpha_beta_x_y(1,Index)+sin_theta_el*Factors_alpha_beta_x_y(2,Index);
        Factors_d_q_x_y(2,1) = -sin_theta_el*Factors_alpha_beta_x_y(1,Index)+cos_theta_el*Factors_alpha_beta_x_y(2,Index);
    
        %Calculation of the voltages per switching state in alpha beta coordinates
        d_q_x_y_voltages_per_switching_state = single(u_dc_link_voltage*Factors_d_q_x_y);
    
        d_voltage_per_switching_state = d_q_x_y_voltages_per_switching_state(1,1);
        q_voltage_per_switching_state = d_q_x_y_voltages_per_switching_state(2,1);
        x_voltage_per_switching_state = d_q_x_y_voltages_per_switching_state(3,1);
        y_voltage_per_switching_state = d_q_x_y_voltages_per_switching_state(4,1);
    

end

== matlab function gm_parallel_phase_voltages_per_switching_state_6_vnl/Phase_voltages_per_switching_state_vnl/Subsystem/MATLAB Function15 ==
  data: theta_el_with_offset input; d_voltage_per_switching_state output; u_dc_link_voltage input; Index input; q_voltage_per_switching_state output; x_voltage_per_switching_state output; y_voltage_per_switching_state output
function [d_voltage_per_switching_state, q_voltage_per_switching_state, x_voltage_per_switching_state, y_voltage_per_switching_state] = fcn(theta_el_with_offset, u_dc_link_voltage, Index)
      
        % Initial condition
            Index = Index+1;

        % Swichtingstates factors alpha beta x y
        Factors_alpha_beta_x_y = single([0	    0.333333333333333	-0.166666666666667	 0.166666666666667;
                                         0	    0                    0.288675134594813	 0.288675134594813;
                                         0	    0.333333333333333	-0.166666666666667	 0.166666666666667;
                                         0	    0	                -0.288675134594813	-0.288675134594813]);
        
        % Park-Transformation of the switchingstates factors
        Factors_d_q_x_y =single(zeros(4,1));
    
        Factors_d_q_x_y(3,1) = Factors_alpha_beta_x_y(3,Index);
        Factors_d_q_x_y(4,1) = Factors_alpha_beta_x_y(4,Index);
    
        cos_theta_el = single(cos(theta_el_with_offset));
        sin_theta_el = single(sin(theta_el_with_offset));
       
        Factors_d_q_x_y(1,1) = cos_theta_el*Factors_alpha_beta_x_y(1,Index)+sin_theta_el*Factors_alpha_beta_x_y(2,Index);
        Factors_d_q_x_y(2,1) = -sin_theta_el*Factors_alpha_beta_x_y(1,Index)+cos_theta_el*Factors_alpha_beta_x_y(2,Index);
    
        %Calculation of the voltages per switching state in alpha beta coordinates
        d_q_x_y_voltages_per_switching_state = single(u_dc_link_voltage*Factors_d_q_x_y);
    
        d_voltage_per_switching_state = d_q_x_y_voltages_per_switching_state(1,1);
        q_voltage_per_switching_state = d_q_x_y_voltages_per_switching_state(2,1);
        x_voltage_per_switching_state = d_q_x_y_voltages_per_switching_state(3,1);
        y_voltage_per_switching_state = d_q_x_y_voltages_per_switching_state(4,1);
    

end

== matlab function gm_parallel_phase_voltages_per_switching_state_6_vnl/Phase_voltages_per_switching_state_vnl/Subsystem/MATLAB Function1 ==
  data: theta_el_with_offset input; d_voltage_per_switching_state output; u_dc_link_voltage input; Index input; q_voltage_per_switching_state output; x_voltage_per_switching_state output; y_voltage_per_switching_state output
function [d_voltage_per_switching_state, q_voltage_per_switching_state, x_voltage_per_switching_state, y_voltage_per_switching_state] = fcn(theta_el_with_offset, u_dc_link_voltage, Index)
      
        % Initial condition
            Index = Index+1;

    
        % Swichtingstates factors alpha beta x y
        Factors_alpha_beta_x_y = single([0	0.333333333333333	-0.166666666666667	 0.166666666666667;
                                         0	0	                 0.288675134594813	 0.288675134594813;
                                         0	0.333333333333333	-0.166666666666667	 0.166666666666667;
                                         0	0	                -0.288675134594813	-0.288675134594813]);
        
        % Park-Transformation of the switchingstates factors
        Factors_d_q_x_y =single(zeros(4,1));
    
        Factors_d_q_x_y(3,1) = Factors_alpha_beta_x_y(3,Index);
        Factors_d_q_x_y(4,1) = Factors_alpha_beta_x_y(4,Index);
    
        cos_theta_el = single(cos(theta_el_with_offset));
        sin_theta_el = single(sin(theta_el_with_offset));
       
        Factors_d_q_x_y(1,1) = cos_theta_el*Factors_alpha_beta_x_y(1,Index)+sin_theta_el*Factors_alpha_beta_x_y(2,Index);
        Factors_d_q_x_y(2,1) = -sin_theta_el*Factors_alpha_beta_x_y(1,Index)+cos_theta_el*Factors_alpha_beta_x_y(2,Index);
    
        %Calculation of the voltages per switching state in alpha beta coordinates
        d_q_x_y_voltages_per_switching_state = single(u_dc_link_voltage*Factors_d_q_x_y);
    
        d_voltage_per_switching_state = d_q_x_y_voltages_per_switching_state(1,1);
        q_voltage_per_switching_state = d_q_x_y_voltages_per_switching_state(2,1);
        x_voltage_per_switching_state = d_q_x_y_voltages_per_switching_state(3,1);
        y_voltage_per_switching_state = d_q_x_y_voltages_per_switching_state(4,1);
    

end

== matlab function gm_parallel_phase_voltages_per_switching_state_6_vnl/Phase_voltages_per_switching_state_vnl/Subsystem/MATLAB Function2 ==
  data: theta_el_with_offset input; d_voltage_per_switching_state output; u_dc_link_voltage input; Index input; q_voltage_per_switching_state output; x_voltage_per_switching_state output; y_voltage_per_switching_state output
function [d_voltage_per_switching_state, q_voltage_per_switching_state, x_voltage_per_switching_state, y_voltage_per_switching_state] = fcn(theta_el_with_offset, u_dc_link_voltage, Index)
      
        % Initial condition
            Index = Index+1;

        % Swichtingstates factors alpha beta x y
        Factors_alpha_beta_x_y = single([-0.455341801261480	-0.122008467928146	-0.622008467928146	-0.288675134594813;
                                         -0.455341801261480	-0.455341801261480	-0.166666666666667	-0.166666666666667;
                                         0.122008467928146	 0.455341801261480	-0.0446581987385205  0.288675134594813;
                                         0.122008467928146	 0.122008467928146	-0.166666666666667	-0.166666666666667]);
        
        % Park-Transformation of the switchingstates factors
        Factors_d_q_x_y =single(zeros(4,1));
    
        Factors_d_q_x_y(3,1) = Factors_alpha_beta_x_y(3,Index);
        Factors_d_q_x_y(4,1) = Factors_alpha_beta_x_y(4,Index);
    
        cos_theta_el = single(cos(theta_el_with_offset));
        sin_theta_el = single(sin(theta_el_with_offset));
       
        Factors_d_q_x_y(1,1) = cos_theta_el*Factors_alpha_beta_x_y(1,Index)+sin_theta_el*Factors_alpha_beta_x_y(2,Index);
        Factors_d_q_x_y(2,1) = -sin_theta_el*Factors_alpha_beta_x_y(1,Index)+cos_theta_el*Factors_alpha_beta_x_y(2,Index);
    
        %Calculation of the voltages per switching state in alpha beta coordinates
        d_q_x_y_voltages_per_switching_state = single(u_dc_link_voltage*Factors_d_q_x_y);
    
        d_voltage_per_switching_state = d_q_x_y_voltages_per_switching_state(1,1);
        q_voltage_per_switching_state = d_q_x_y_voltages_per_switching_state(2,1);
        x_voltage_per_switching_state = d_q_x_y_voltages_per_switching_state(3,1);
        y_voltage_per_switching_state = d_q_x_y_voltages_per_switching_state(4,1);
    

end

== matlab function gm_parallel_phase_voltages_per_switching_state_6_vnl/Phase_voltages_per_switching_state_vnl/Subsystem/MATLAB Function3 ==
  data: theta_el_with_offset input; d_voltage_per_switching_state output; u_dc_link_voltage input; Index input; q_voltage_per_switching_state output; x_voltage_per_switching_state output; y_voltage_per_switching_state output
function [d_voltage_per_switching_state, q_voltage_per_switching_state, x_voltage_per_switching_state, y_voltage_per_switching_state] = fcn(theta_el_with_offset, u_dc_link_voltage, Index)
      
        % Initial condition
            Index = Index+1;

    
        % Swichtingstates factors alpha beta x y
        Factors_alpha_beta_x_y = single([-0.288675134594813	 0.0446581987385205  -0.455341801261480	  -0.122008467928146;
                                         -0.166666666666667	-0.166666666666667	  0.122008467928146	   0.122008467928146;
                                         0.288675134594813	 0.622008467928146	  0.122008467928146	   0.455341801261480;
                                         -0.166666666666667	-0.166666666666667	 -0.455341801261480	  -0.455341801261480]);
        
        % Park-Transformation of the switchingstates factors
        Factors_d_q_x_y =single(zeros(4,1));
    
        Factors_d_q_x_y(3,1) = Factors_alpha_beta_x_y(3,Index);
        Factors_d_q_x_y(4,1) = Factors_alpha_beta_x_y(4,Index);
    
        cos_theta_el = single(cos(theta_el_with_offset));
        sin_theta_el = single(sin(theta_el_with_offset));
       
        Factors_d_q_x_y(1,1) = cos_theta_el*Factors_alpha_beta_x_y(1,Index)+sin_theta_el*Factors_alpha_beta_x_y(2,Index);
        Factors_d_q_x_y(2,1) = -sin_theta_el*Factors_alpha_beta_x_y(1,Index)+cos_theta_el*Factors_alpha_beta_x_y(2,Index);
    
        %Calculation of the voltages per switching state in alpha beta coordinates
        d_q_x_y_voltages_per_switching_state = single(u_dc_link_voltage*Factors_d_q_x_y);
    
        d_voltage_per_switching_state = d_q_x_y_voltages_per_switching_state(1,1);
        q_voltage_per_switching_state = d_q_x_y_voltages_per_switching_state(2,1);
        x_voltage_per_switching_state = d_q_x_y_voltages_per_switching_state(3,1);
        y_voltage_per_switching_state = d_q_x_y_voltages_per_switching_state(4,1);
    

end

== matlab function gm_parallel_phase_voltages_per_switching_state_6_vnl/Phase_voltages_per_switching_state_vnl/Subsystem/MATLAB Function4 ==
  data: theta_el_with_offset input; d_voltage_per_switching_state output; u_dc_link_voltage input; Index input; q_voltage_per_switching_state output; x_voltage_per_switching_state output; y_voltage_per_switching_state output
function [d_voltage_per_switching_state, q_voltage_per_switching_state, x_voltage_per_switching_state, y_voltage_per_switching_state] = fcn(theta_el_with_offset, u_dc_link_voltage, Index)
      
        % Initial condition
            Index = Index+1;

    
        % Swichtingstates factors alpha beta x y
        Factors_alpha_beta_x_y = single([0.122008467928146	 0.455341801261480	-0.0446581987385205  0.288675134594813;
                                         -0.455341801261480	-0.455341801261480	-0.166666666666667	-0.166666666666667;
                                         -0.455341801261480	-0.122008467928146	-0.622008467928146	-0.288675134594813;
                                         0.122008467928146	 0.122008467928146	-0.166666666666667	-0.166666666666667]);
        
        % Park-Transformation of the switchingstates factors
        Factors_d_q_x_y =single(zeros(4,1));
    
        Factors_d_q_x_y(3,1) = Factors_alpha_beta_x_y(3,Index);
        Factors_d_q_x_y(4,1) = Factors_alpha_beta_x_y(4,Index);
    
        cos_theta_el = single(cos(theta_el_with_offset));
        sin_theta_el = single(sin(theta_el_with_offset));
       
        Factors_d_q_x_y(1,1) = cos_theta_el*Factors_alpha_beta_x_y(1,Index)+sin_theta_el*Factors_alpha_beta_x_y(2,Index);
        Factors_d_q_x_y(2,1) = -sin_theta_el*Factors_alpha_beta_x_y(1,Index)+cos_theta_el*Factors_alpha_beta_x_y(2,Index);
    
        %Calculation of the voltages per switching state in alpha beta coordinates
        d_q_x_y_voltages_per_switching_state = single(u_dc_link_voltage*Factors_d_q_x_y);
    
        d_voltage_per_switching_state = d_q_x_y_voltages_per_switching_state(1,1);
        q_voltage_per_switching_state = d_q_x_y_voltages_per_switching_state(2,1);
        x_voltage_per_switching_state = d_q_x_y_voltages_per_switching_state(3,1);
        y_voltage_per_switching_state = d_q_x_y_voltages_per_switching_state(4,1);
    

end
